simulink model "car_sim_for_student_r2015"  (R2022a)
settings: Solver=FixedStepAuto  StartTime=0.0  StopTime=40  FixedStep=0.001  RelTol=1e-3
InitFcn:
  | run lqr_nums.m
StopFcn:
  | save(['结果展示/out_simout',pathnums,'.mat'],'out')
values from neighbouring files (symbols this model uses):
  k = lqr(A,B,Q,R)    [lqr_nums.m]
  map = imresize(before_map,s)    [Generate_Miniature_Path.m]    (also in Smooth_Path.m = ~map; make_GIF.m = map_from_initcallback)
  out = display_car(map_coord,phi,l,w,map,out)    [make_GIF.m]
  trajSYSU = trajSYSU/100    [Smooth_Path.m]
undefined symbols (not defined in the file or in its folder): gray
libraries: simulink x2, slpidlib x1
settings Model: Creator=Manny  LastModifiedBy=翎雨
settings OptimizationCC: LifeSpan=inf
settings DebuggingCC: UnconnectedInputMsg=warning  UnconnectedOutputMsg=warning  UnconnectedLineMsg=warning  SFExecutionAtInitializationDiag=none  SFMachineParentedDataDiag=warning  ArithmeticOperatorsInVariantConditions=warning
settings SFSimCC: CustomCodeUndefinedFunction=UseInterfaceOnly
settings CodeAppCC: StateflowObjectComments=on

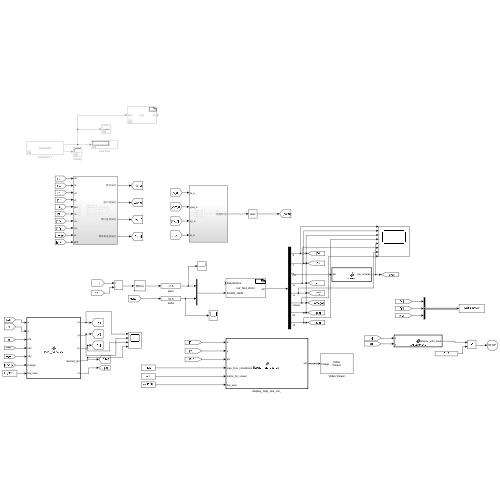
[thumbnail: Simulink's stored preview of the top-level diagram]
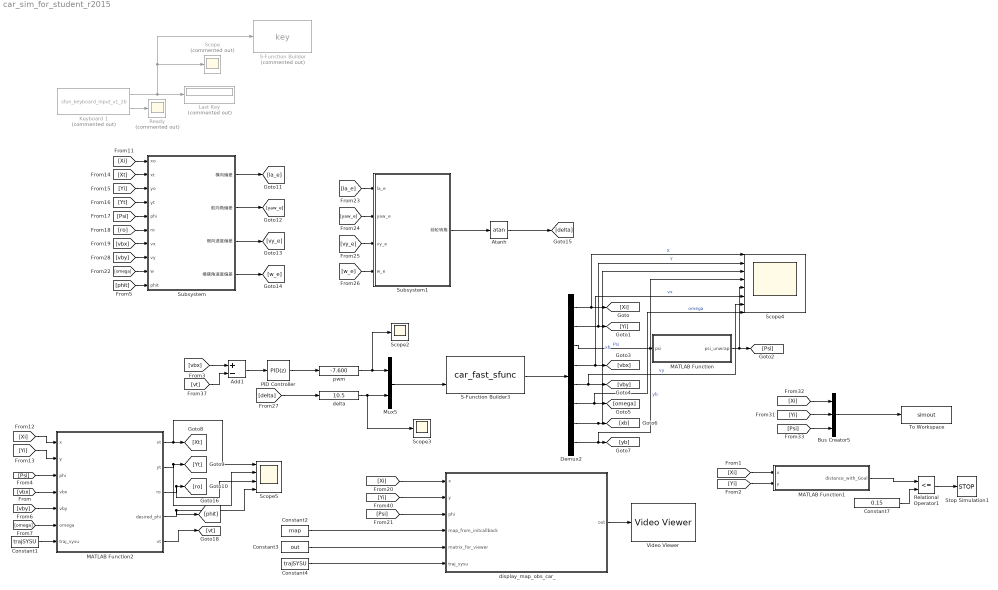
== system car_sim_for_student_r2015 ==
  Add1 : Sum  Inputs=+-
  Atanh : Trigonometry  Operator=atan
  Bus Creator5 : BusCreator  Inputs=3
  Constant1 : Constant  Value=trajSYSU
  Constant2 : Constant  Value=map
  Constant3 : Constant  Value=out
  Constant4 : Constant  Value=trajSYSU
  Constant7 : Constant  Value=0.15
  Demux2 : Demux  Outputs=8
  Keyboard 1 : M-S-Function  Commented=on  FunctionName=sfun_keyboard_input_v1_2b  mask(Keyboard Input){}
      mask help: Keyboard Input
      mask Display: fprintf('Keyboard');
  Last Key : Display  Commented=on
  MATLAB Function : MATLAB Function  TreatAsAtomicUnit=on
  MATLAB Function1 : MATLAB Function  TreatAsAtomicUnit=on
  MATLAB Function2 : MATLAB Function  TreatAsAtomicUnit=on
  Mux5 : Mux  Inputs=2
  PID Controller : slpidlib/PID Controller  Controller=PID  Form=Parallel  TimeDomain=Discrete-time  UseExternalTs=off  SampleTime=-1  IntegratorMethod=Forward Euler  FilterMethod=Forward Euler  ControllerParametersSource=internal  P=2.5  I=1.2  UseKiTs=off  D=0.2  N=100  UseFilter=on  TunerSelectOption=Transfer Function Based (PID Tuner App)  InitialConditionSource=internal  InitialConditionForIntegrator=0  InitialConditionForFilter=0  DifferentiatorICPrevScaledInput=0  ExternalReset=none  TrackingMode=off  Kt=1  LimitOutput=off  SatLimitsSource=internal  UpperSaturationLimit=inf  LowerSaturationLimit=-inf  LinearizeAsGain=on  AntiWindupMode=none  Kb=1  POutMin=[]  POutMax=[]  IOutMin=[]  IOutMax=[]  DOutMin=[]  DOutMax=[]  NOutMin=[]  NOutMax=[]  SumOutMin=[]  SumOutMax=[]  SaturationOutMin=[]  SaturationOutMax=[]  PParamMin=[]  PParamMax=[]  IParamMin=[]  IParamMax=[]  DParamMin=[]  DParamMax=[]  NParamMin=[]  NParamMax=[]  KbParamMin=[]  KbParamMax=[]  KtParamMin=[]  KtParamMax=[]  KbOutMin=[]  KbOutMax=[]  KtOutMin=[]  KtOutMax=[]  IntegratorOutMin=[]  IntegratorOutMax=[]  FilterOutMin=[]  FilterOutMax=[]  SumI1OutMin=[]  SumI1OutMax=[]  SumI2OutMin=[]  SumI2OutMax=[]  SumI3OutMin=[]  SumI3OutMax=[]  SumI4OutMin=[]  SumI4OutMax=[]  SumDOutMin=[]  SumDOutMax=[]  DifferentiatorOutMin=[]  DifferentiatorOutMax=[]  FilterDiffOutCoefMin=[]  FilterDiffOutCoefMax=[]  ReciprocalOutMin=[]  ReciprocalOutMax=[]  SumDenOutMin=[]  SumDenOutMax=[]  SumNumOutMin=[]  SumNumOutMax=[]  DivideOutMin=[]  DivideOutMax=[]  UdiffTsProdOutMin=[]  UdiffTsProdOutMax=[]  NTsProdOutMin=[]  NTsProdOutMax=[]  UintegralTsProdOutMin=[]  UintegralTsProdOutMax=[]  UngainTsProdOutMin=[]  UngainTsProdOutMax=[]  IntegratorContinuousStateAttributes=''  IntegratorStateMustResolveToSignalObject=off  IntegratorRTWStateStorageClass=Auto  FilterContinuousStateAttributes=''  FilterStateMustResolveToSignalObject=off  FilterRTWStateStorageClass=Auto  ParallelPVariant=InternalParameters  IdealPVariant=Disabled  IVariant=InternalParameters  DVariant=InternalParameters  IntegratorVariant=Discrete  SatVariant=Disabled  AWVariant=Passthrough  PCopyVariant=Disabled  TRVariant=Disabled  FdbkBlocksVariant=Forward  IdealPFdbkVariant=Disabled  SatFdbkVariant=Disabled  DerivativeFilterVariant=ForwardEulerFilter  NVariant=InternalParameters  NCopyVariant=Disabled  FilterICVariant=InternalICsFilter  IntegratorICVariant=InternalICs  ExternalResetVariant=Disabled  TRSumVariant=Passthrough  SumFdbkVariant=Disabled  SumVariant=Sum_PID  TsampFilterVariant=InternalTs  TsampNgainVariant=Passthrough  TsampIntegralVariant=Passthrough  ExternalSaturationOutDataTypeStr=Inherit: Same as second input  aMode=0
  Ready : Scope  Commented=on
  Relational Operator1 : RelationalOperator  Operator=<=  OutDataTypeStr=boolean  InputSameDT=off
  S-Function Builder : S-Function  Commented=on  FunctionName=key  SFunctionModules=key_wrapper  SFunctionDeploymentMode=off  EnableBusSupport=off  mask(S-Function Builder){}
      mask help: Simulink:masks:SFunctionBuilder_MD
      mask init:
      | val = [[.9  0.75 0.75 1 1 .9 .9 1]',[1 1 0.75 0.75 .9 .9 1 .9]'];try , sys = get_param(gcb,'SfunBuilderFcnName');if isempty(sys), sys = get_param(gcb,'FunctionName'); end,catch, sys = get_param(gcb,'FunctionName'); end
      settings: CopyFcn=set_param(gcbh,'LinkStatus','none')  OpenFcn=sfunctionwizard(gcbh)
      mask Display:
      | plot(val(:,1),val(:,2))
      | disp(sys)
      | port_label('input',1,'key')
      | port_label('output',1,'y0')
  S-Function Builder3 : S-Function  FunctionName=car_fast_sfunc  SFunctionModules=car_fast_sfunc_wrapper  SFunctionDeploymentMode=off  EnableBusSupport=off  mask(S-Function Builder){}
      mask help: Simulink:masks:SFunctionBuilder_MD
      mask init: same as car_sim_for_student_r2015/S-Function Builder
      settings: CopyFcn=set_param(gcbh,'LinkStatus','none')  OpenFcn=sfunctionwizard(gcbh)
      mask Display:
      | plot(val(:,1),val(:,2))
      | disp(sys)
      | port_label('input',1,'disturbance')
      | port_label('input',2,'throttle_delta')
      | port_label('output',1,'y0')
  Scope : Scope  Commented=on
  Scope2 : Scope
  Scope3 : Scope
  Scope4 : Scope  NumInputPorts=8
  Scope5 : Scope  NumInputPorts=4
  Stop Simulation1 : Stop
  Subsystem : Subsystem
  Subsystem1 : Subsystem
  To Workspace : ToWorkspace  VariableName=simout  SaveFormat=Timeseries  SampleTime=-1
  Video Viewer : VideoViewer  colormapValue=gray(256)  FigPos=[1 822 1536 724.8]
  delta : simulink/Math Operations/Slider Gain  gain=10.5  low=-20  high=20
  display_map_obs_car_ : MATLAB Function  TreatAsAtomicUnit=on
  pwm : simulink/Math Operations/Slider Gain  gain=-7.600  low=-20  high=20
  wires:
  S-Function Builder3/1 -> Demux2/1
  Demux2/2 -> Scope4/2, [Yi]  "Y"
  Demux2/3 -> MATLAB Function/1(psi)  "Psi"
  Demux2/4 -> Scope4/6, [vbx]  "vx"
  Demux2/5 -> Scope4/7, [vby]  "vy"
  Demux2/6 -> Scope4/8, [omega]  "omega"
  Demux2/7 -> Scope4/3, [xb]  "xb"
  Demux2/8 -> Scope4/4, [yb]  "yb"
  MATLAB Function/1(psi_unwrap) -> Scope4/5, [Psi]
  [Yi] -> display_map_obs_car_/2(y)
  [Xi] -> display_map_obs_car_/1(x)
  [Psi] -> display_map_obs_car_/3(phi)
  display_map_obs_car_/1(out) -> Video Viewer/1
  Constant2/1 -> display_map_obs_car_/4(map_from_initcallback)
  Demux2/1 -> Scope4/1, [Xi]  "X"
  Constant3/1 -> display_map_obs_car_/5(matrix_for_viewer)
  pwm/1 -> Scope2/1, Mux5/1
  Keyboard 1/1 -> S-Function Builder/1, Scope/1, Last Key/1
  Keyboard 1/2 -> Ready/1
  [Yi] -> Bus Creator5/2
  Bus Creator5/1 -> To Workspace/1
  [Psi] -> Bus Creator5/3
  [Xi] -> Bus Creator5/1
  Mux5/1 -> S-Function Builder3/2
  [Xi] -> MATLAB Function1/1(x)
  MATLAB Function1/1(distance_with_Goal) -> Relational Operator1/1
  Relational Operator1/1 -> Stop Simulation1/1
  Constant7/1 -> Relational Operator1/2
  [Yi] -> MATLAB Function1/2(y)
  [Psi] -> MATLAB Function2/3(phi)
  Constant4/1 -> display_map_obs_car_/6(traj_sysu)
  [vbx] -> MATLAB Function2/4(vbx)
  [omega] -> MATLAB Function2/6(omega)
  [vby] -> MATLAB Function2/5(vby)
  delta/1 -> Scope3/1, Mux5/2
  [Yi] -> MATLAB Function2/2(y)
  Constant1/1 -> MATLAB Function2/7(traj_sysu)
  [Xi] -> MATLAB Function2/1(x)
  Add1/1 -> PID Controller/1
  PID Controller/1 -> pwm/1
  [vbx] -> Add1/1
  [vt] -> Add1/2
  MATLAB Function2/1(xt) -> Scope5/1, [Xt]
  MATLAB Function2/2(yt) -> Scope5/2, [Yt]
  MATLAB Function2/3(ro) -> Scope5/3, [ro]
  [Xi] -> Subsystem/1(xo)
  [Xt] -> Subsystem/2(xt)
  [Yi] -> Subsystem/3(yo)
  [Yt] -> Subsystem/4(yt)
  [Psi] -> Subsystem/5(phi)
  [ro] -> Subsystem/6(ro)
  [vbx] -> Subsystem/7(vx)
  Subsystem/1(横向偏差) -> [la_e]
  Subsystem/2(航向角偏差) -> [yaw_e]
  Subsystem/3(侧向速度偏差) -> [vy_e]
  Subsystem/4(横摆角速度偏差) -> [w_e]
  [la_e] -> Subsystem1/1(la_e)
  [yaw_e] -> Subsystem1/2(yaw_e)
  [vy_e] -> Subsystem1/3(vy_e)
  [w_e] -> Subsystem1/4(w_e)
  [omega] -> Subsystem/9(w)
  [vby] -> Subsystem/8(vy)
  MATLAB Function2/4(desired_phi) -> [phit], Scope5/4
  [phit] -> Subsystem/10(phit)
  MATLAB Function2/5(vt) -> [vt]
  Subsystem1/1(前轮转角) -> Atanh/1
  Atanh/1 -> [delta]
  [delta] -> delta/1

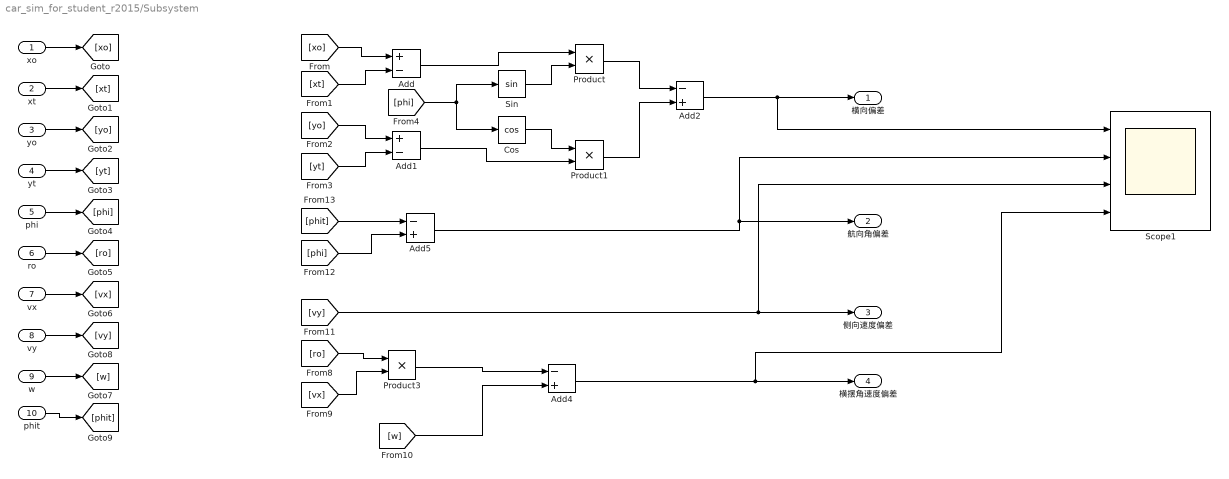
== system car_sim_for_student_r2015/Subsystem ==
  xo : Inport
  xt : Inport  Port=2
  yo : Inport  Port=3
  yt : Inport  Port=4
  phi : Inport  Port=5
  ro : Inport  Port=6
  vx : Inport  Port=7
  vy : Inport  Port=8
  w : Inport  Port=9
  phit : Inport  Port=10
  Add : Sum  Inputs=+-
  Add1 : Sum  Inputs=+-
  Add2 : Sum  Inputs=-+
  Add4 : Sum  Inputs=-+
  Add5 : Sum  Inputs=-+
  Cos : Trigonometry  Operator=cos
  Product : Product
  Product1 : Product
  Product3 : Product
  Scope1 : Scope  NumInputPorts=4
  Sin : Trigonometry
  横向偏差 : Outport
  航向角偏差 : Outport  Port=2
  侧向速度偏差 : Outport  Port=3
  横摆角速度偏差 : Outport  Port=4
  wires:
  xo/1 -> [xo]
  xt/1 -> [xt]
  yo/1 -> [yo]
  yt/1 -> [yt]
  phi/1 -> [phi]
  ro/1 -> [ro]
  vx/1 -> [vx]
  [xo] -> Add/1
  [xt] -> Add/2
  [yo] -> Add1/1
  [yt] -> Add1/2
  [phi] -> Sin/1, Cos/1
  Add/1 -> Product/1
  Sin/1 -> Product/2
  Product/1 -> Add2/1
  Cos/1 -> Product1/1
  Add1/1 -> Product1/2
  Product1/1 -> Add2/2
  Add2/1 -> Scope1/1, 横向偏差/1
  [ro] -> Product3/1
  Product3/1 -> Add4/1
  [w] -> Add4/2
  Add4/1 -> Scope1/4, 横摆角速度偏差/1
  [vy] -> Scope1/3, 侧向速度偏差/1
  w/1 -> [w]
  vy/1 -> [vy]
  phit/1 -> [phit]
  Add5/1 -> Scope1/2, 航向角偏差/1
  [phit] -> Add5/1
  [phi] -> Add5/2
  [vx] -> Product3/2

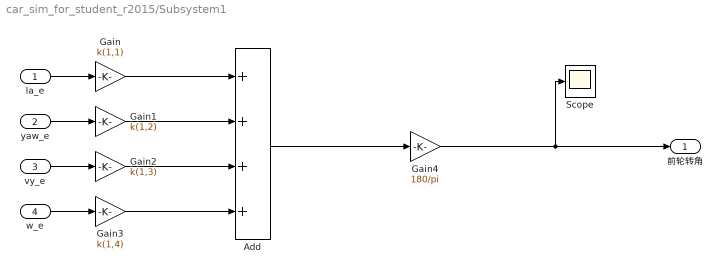
== system car_sim_for_student_r2015/Subsystem1 ==
  la_e : Inport
  yaw_e : Inport  Port=2
  vy_e : Inport  Port=3
  w_e : Inport  Port=4
  Add : Sum  Inputs=++++
  Gain : Gain  Gain=k(1,1)
  Gain1 : Gain  Gain=k(1,2)
  Gain2 : Gain  Gain=k(1,3)
  Gain3 : Gain  Gain=k(1,4)
  Gain4 : Gain  Gain=180/pi
  Scope : Scope
  前轮转角 : Outport
  wires:
  la_e/1 -> Gain/1
  yaw_e/1 -> Gain1/1
  vy_e/1 -> Gain2/1
  w_e/1 -> Gain3/1
  Gain/1 -> Add/1
  Gain1/1 -> Add/2
  Gain2/1 -> Add/3
  Gain3/1 -> Add/4
  Add/1 -> Gain4/1
  Gain4/1 -> Scope/1, 前轮转角/1

== matlab function car_sim_for_student_r2015/MATLAB Function1 ==
  data: x input; distance_with_Goal output; y input
function distance_with_Goal = cal_distance(x,y)
distance_with_Goal=sqrt((x-11.3)*(x-11.3)+(y-4.5)*(y-4.5));

== matlab function car_sim_for_student_r2015/display_map_obs_car_ ==
  settings: updateMethod=DISCRETE
  data: x input; y input; phi input; out output size=600,1200,3; map_from_initcallback input size=600,1200; matrix_for_viewer input; traj_sysu input
function out = display_map_obs_car_(x,y,phi,map_from_initcallback,matrix_for_viewer,traj_sysu)
    persistent data;
    persistent times;
    if isempty(data)
        times=1;
    else
        times=times+1;
    end

    % 地图长12m 宽6m   车长0.12 车宽0.06
    resolution = 0.01;
    map_long=12;
    map_wide=6;

    car_long=0.12;
    car_wide=0.06;

%     % 可视化地图
%     figure;
%     imagesc(map);%imagesc 可以将矩阵或数组的值映射到颜色图像中
%     colormap(flipud(gray));%colormap 将数据值映射到颜色空间中 colormap(flipud(gray)) 来设置颜色映射表为灰度图像。
    map=map_from_initcallback;    
    out=matrix_for_viewer;
    number_path=size(traj_sysu,2);
    for tmp=1:number_path
        traj_sysu_index=real2map([traj_sysu(1,tmp),traj_sysu(2,tmp)],map_wide,resolution);
        out(round(traj_sysu_index(1)+1/2),round(traj_sysu_index(2)+1/2),:)=[0,0,0];
    end
    x_now=x;%m  real视野坐标系,横着往右
    y_now=y;%m  real视野坐标系,竖着往上
    map_coord=real2map([x_now,y_now],map_wide,resolution);
    if isempty(data)
        data = zeros(99999, 2);
    else
        data(round(times/10)+1,:) = [map_coord(1),map_coord(2)];
        for times_disp_tmp=1:round(times/10)
            tmp_Data=data(times_disp_tmp,:);
            tmp_Data_next=data(times_disp_tmp+1,:);
%             out(round(tmp_Data(1,1)+1/2),round(tmp_Data(1,2)+1/2),:)=[0,0,1];

    
            vector=tmp_Data_next-tmp_Data;
            for t=0:0.025:1
                    new_point=tmp_Data+t*vector;
                    out(round(new_point(1)+1/2),round(new_point(2)+1/2),:)=[0,0,1];
                    out(round(new_point(1)+1/2),round(new_point(2)+1/2)-1,:)=[0,0,1];
                    out(round(new_point(1)+1/2),round(new_point(2)+1/2)+1,:)=[0,0,1];
            end

        end
    end



   
%     occ_or_not=get_occ_or_not(map_coord,map,resolution)
    occ_or_not=get_occ_or_not_Real([x_now,y_now],map_wide,map,resolution);
    l = car_long / resolution;
    w = car_wide / resolution;
    phi = phi; 




out=display_car(map_coord,phi,l,w,map,out);

%     axis equal;
%     axis off;
end

function occ_or_not=get_occ_or_not_Real(x_y,map_wide,map,resolution)
%round四舍五入 
map_coord=real2map(x_y,map_wide,resolution);
if(round(map_coord(1)+1/2)<1) ||(round(map_coord(1)+1/2)>600) ||(round(map_coord(2)+1/2)<1) ||(round(map_coord(2)+1/2)>1200)
    x_y
    disp('out of map');
end
 occ_or_not=map(round(map_coord(1)+1/2),round(map_coord(2)+1/2));
end
function occ_or_not=get_occ_or_not_map(map_coord,map,resolution)
%round四舍五入 
if(round(map_coord(1)+1/2)<1) ||(round(map_coord(1)+1/2)>600) ||(round(map_coord(2)+1/2)<1) ||(round(map_coord(2)+1/2)>1200)
    disp('out of map');
end
 occ_or_not=map(round(map_coord(1)+1/2),round(map_coord(2)+1/2));
end
function map_coord=real2map(x_y,map_wide,resolution)
    %地图向下是正x 向右是正y，
    % 因此在map上显示赛道小车障碍物的时候map_y直接取real世界的x, map_x需要把real_y反向并弄个静差
    map_coord=zeros(1,2);
    map_coord(1)=map_wide/ resolution-x_y(2)/ resolution;
    map_coord(2)=x_y(1)/ resolution ;
end

function matrix_for_viewer_new=display_car(map_coord,phi,l,w,map,matrix_for_viewer)
    %display是向右是x正，向下是y正
    pts = [
        map_coord(1)- [sin(phi)*l-cos(phi)*w, sin(phi)*l+cos(phi)*w,-sin(phi)*l+cos(phi)*w,-sin(phi)*l-cos(phi)*w]
        map_coord(2) + [cos(phi)*l+sin(phi)*w, cos(phi)*l-sin(phi)*w,-cos(phi)*l-sin(phi)*w,-cos(phi)*l+sin(phi)*w]
        
    ];
    map_index1=[round(pts(1,1)+1/2),round(pts(2,1)+1/2)];
    map_index2=[round(pts(1,2)+1/2),round(pts(2,2)+1/2)];
    map_index3=[round(pts(1,3)+1/2),round(pts(2,3)+1/2)];
    map_index4=[round(pts(1,4)+1/2),round(pts(2,4)+1/2)];

    matrix_for_viewer_new=matrix_for_viewer;
    %凸包，边缘线无碰撞则整体无碰撞
    have_somewhere_occ=0;
    vector_A_B=[map_index2(1)-map_index1(1),map_index2(2)-map_index1(2)];
    vector_A_D=[map_index4(1)-map_index1(1),map_index4(2)-map_index1(2)];
    for t1=0:0.025:1
        for t2=0:0.025:1
            new_point=map_index1+t1*vector_A_B+t2*vector_A_D;
            matrix_for_viewer_new(round(new_point(1)+0.5),round(new_point(2)+0.5),:)=[1,0,0];
            occ_or_not=map(round(new_point(1)+0.5),round(new_point(2)+0.5));
            if(occ_or_not==1)
               have_somewhere_occ=1;
           end
        end
    end
    if(have_somewhere_occ==1)
%         disp("collision!!");
    end
end

== matlab function car_sim_for_student_r2015/MATLAB Function ==
  data: psi input; psi_unwrap output
function psi_unwrap= unwrap(psi)

while ( psi > pi)
    psi = psi - 2*pi;
end

while( psi <= -pi)
    psi = psi + 2*pi;
end
psi_unwrap = psi;

== matlab function car_sim_for_student_r2015/MATLAB Function2 ==
  data: x input; xt output; y input; yt output; phi input; vbx input; vby input; omega input; traj_sysu input; ro output; desired_phi output; vt output
function [xt,yt,ro,desired_phi,vt] = Ideal_trajectory(x, y, phi, vbx, vby, omega,traj_sysu)
    % 寻找最近的路径点
    len=size(traj_sysu,2);
    distances = (traj_sysu(1,:) - x).^2 + (traj_sysu(2,:) - y).^2;
    [~, nearest_index] = min(distances);
    % 计算最近路径点的方向角和曲率
    xt=traj_sysu(1, min(nearest_index+1,len));
    yt=traj_sysu(2, min(nearest_index+1,len));
    desired_phi = traj_sysu(3, min(nearest_index+1,len));
    if abs(phi-desired_phi)>pi*3/2
        desired_phi=phi;
    end
    ro = traj_sysu(4, min(nearest_index+1,len));
    ro_max=max(abs(traj_sysu(4, max(1,nearest_index-5):min(nearest_index+5,len))));
    if  ro_max<0.5
        vt=4;
    else
        vt=min(max(1,abs(omega/ro_max)),2.5);
    end
end
